simulink model "ex4"  (R2020b)
settings: Solver=VariableStepAuto  StartTime=0.0  StopTime=10.0  MaxStep=0.001  RelTol=1e-3
settings Model: Creator=drart  LastModifiedBy=drart

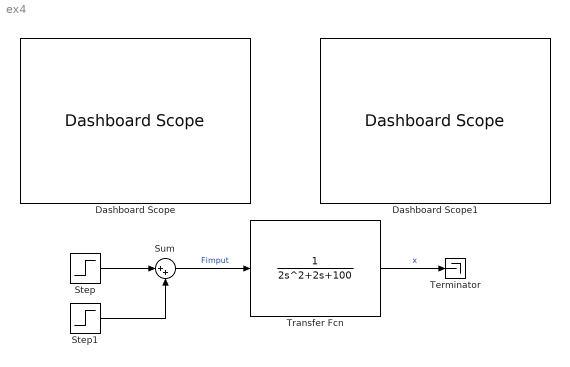
== system ex4 ==
  Dashboard Scope : DashboardScope
  Dashboard Scope1 : DashboardScope
  Step : Step  Time=0  After=50  SampleTime=0
  Step1 : Step  Time=5  After=-50  SampleTime=0
  Sum : Sum  Inputs=|++
  Terminator : Terminator
  Transfer Fcn : TransferFcn  Denominator=[2 2 100]
  wires:
  Step/1 -> Sum/1
  Step1/1 -> Sum/2
  Sum/1 -> Transfer Fcn/1  "Fimput"
  Transfer Fcn/1 -> Terminator/1  "x"
